simulink model "Leg_4DOF_cT_noise_HGOFeedback"  (R2017a)
settings: Solver=FixedStepAuto  StartTime=0.0  StopTime=4  FixedStep=simulation_step  MaxStep=1e-2  RelTol=1e-3  EnableMultiTasking=on
values from neighbouring files (symbols this model uses):
  Ar = [zeros(4) eye(4); zeros(4) zeros(4)]    [Init_HGO.m]
  beta = 10    [Init_4DOF_cT_noise_HGOFeedback.m]
  BodyContact = [ 4 4 ]    [Init_4DOF_cT_noise_HGOFeedback.m]
  BodyContactPositions = [ contact_point_h, contact_point_t ]    [Init_4DOF_cT_noise_HGOFeedback.m]
  Br = [zeros(4); eye(4)]    [Init_HGO.m]
  Cr = [eye(4) zeros(4)]    [Init_HGO.m]
  dqInit = [ 0 0 0 0 ]'    [Init_4DOF_cT_noise_HGOFeedback.m]
  G = g*ez    [Init_4DOF_cT_noise_HGOFeedback.m]
  G_ctrl = g*ez    [Init_4DOF_cT_noise_HGOFeedback.m]
  h = [ ez -ey -ey -ey ]    [Init_4DOF_cT_noise_HGOFeedback.m]
  h_ctrl = h_ctrl.*param_error    [Init_4DOF_cT_noise_HGOFeedback.m]
  Hmu = [eye(4)/Mu zeros(4); zeros(4) eye(4)/Mu^2]    [Init_HGO.m]
  Inertia = [ I_base I_hip I_thigh I_shin I_foot ]    [Init_4DOF_cT_noise_HGOFeedback.m]
  Inertia_ctrl = Inertia_ctrl.*param_error    [Init_4DOF_cT_noise_HGOFeedback.m]
  joint_type = [ 1 0 0 0 ]    [Init_4DOF_cT_noise_HGOFeedback.m]
  k_b = 5000    [Init_4DOF_cT_noise_HGOFeedback.m]
  Kd = kd*eye(n)    [Init_4DOF_cT_noise_HGOFeedback.m]
  Ki = ki*eye(n)    [Init_4DOF_cT_noise_HGOFeedback.m]
  Kp = kp*eye(n)    [Init_4DOF_cT_noise_HGOFeedback.m]
  L = [ l_base_hip l_hip_thigh l_thigh_shin l_shin_foot ]    [Init_4DOF_cT_noise_HGOFeedback.m]
  L_ctrl = L_ctrl.*param_error    [Init_4DOF_cT_noise_HGOFeedback.m]
  L_hgo = [2*eye(4);6*eye(4)]    [Init_HGO.m]
  Mass = [ mass_base mass_hip mass_thigh mass_shin mass_foot ]    [Init_4DOF_cT_noise_HGOFeedback.m]
  Mass_ctrl = Mass_ctrl.*param_error    [Init_4DOF_cT_noise_HGOFeedback.m]
  qInit = [ 0.0216 0.5675 -0.13 -0.39 ]'    [Init_4DOF_cT_noise_HGOFeedback.m]
  R = [ r_base r_hip r_thigh r_shin r_foot ]    [Init_4DOF_cT_noise_HGOFeedback.m]
  R_ctrl = R_ctrl.*param_error    [Init_4DOF_cT_noise_HGOFeedback.m]
  s_z = 2    [Init_4DOF_cT_noise_HGOFeedback.m]
  simulation_step = 1e-4    (= 0.0001)    [Init_4DOF_cT_noise_HGOFeedback.m]
  step_period = t(end)    [Init_4DOF_cT_noise_HGOFeedback.m]
  tau = 0.001    [Init_4DOF_cT_noise_HGOFeedback.m]
undefined symbols (not defined in the file or in its folder): A, Fstate0, magnitude, offset, w
undefined symbols (not defined in the file): window_size
libraries: simulink x1
settings Model: Creator=Ultron  LastModifiedBy=ignacio
settings DataIOCC: LimitDataPoints=on  SaveFormat=Array
settings OptimizationCC: LifeSpan=inf
settings DebuggingCC: SFUnexpectedBacktrackingDiag=warning  SFNoUnconditionalDefaultTransitionDiag=warning  SFExecutionAtInitializationDiag=none
settings HardwareCC: ProdBitPerPointer=32  ProdBitPerSizeT=32  ProdBitPerPtrDiffT=32  ProdLargestAtomicFloat=None  ProdIntDivRoundTo=Undefined  ProdEndianess=Unspecified  ProdWordSize=32  ProdHWDeviceType=32-bit Generic
settings ModelReferenceCC: PropagateSignalLabelsOutOfModel=off
settings GRTTargetCC: TargetLangStandard=C89/C90 (ANSI)  GeneratePreprocessorConditionals=Disable all
settings ConfigComp: CovMetricSettings=dw  CovHtmlReporting=on  CovSaveCumulativeToWorkspaceVar=on  CovSaveSingleToWorkspaceVar=on  CovExternalEMLEnable=off

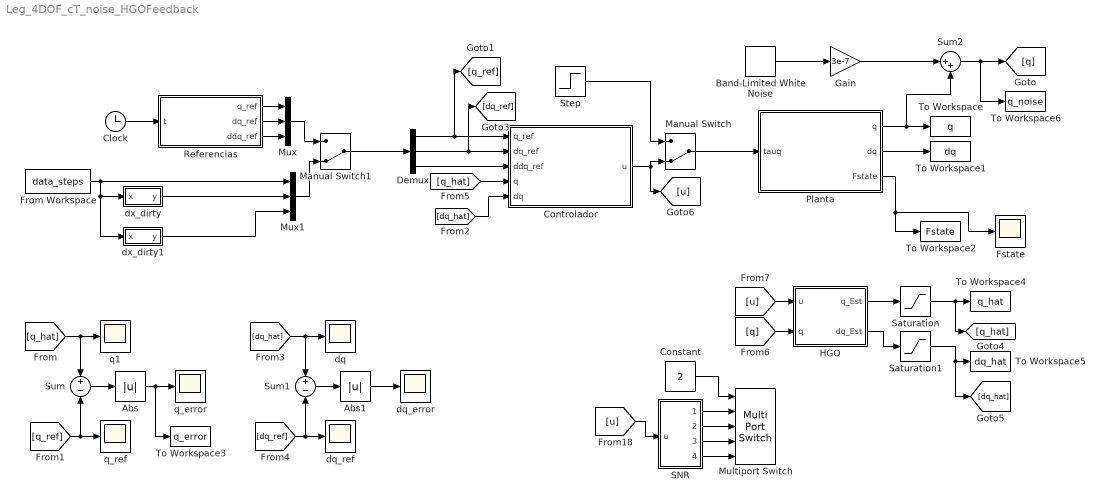
== system Leg_4DOF_cT_noise_HGOFeedback ==
  Abs : Abs
  Abs1 : Abs
  Band-Limited White Noise : simulink/Sources/Band-Limited White Noise  Cov=[0.1]  Ts=simulation_step  seed=[23341]
  Clock : Clock
  Constant : Constant  Value=2
  Controlador : Subsystem
  Demux : Demux  Outputs=3
  From Workspace : FromWorkspace  VariableName=data_steps  SampleTime=0
  Fstate : Scope
  Gain : Gain  Gain=3e-7
  HGO : Subsystem
  Manual Switch : ManualSwitch  CurrentSetting=0
  Manual Switch1 : ManualSwitch  CurrentSetting=0
  Multiport Switch : MultiPortSwitch  Inputs=4
  Mux : Mux  Inputs=3
  Mux1 : Mux  Inputs=3
  Planta : Subsystem
  Referencias : MATLAB Function  TreatAsAtomicUnit=on
  SNR : Subsystem
  Saturation : Saturate  UpperLimit=6*pi  LowerLimit=-6*pi
  Saturation1 : Saturate  UpperLimit=6*pi  LowerLimit=-6*pi
  Step : Step  Before=[0;0;0;0]  After=[0;0;0;0]  SampleTime=0
  Sum : Sum  Inputs=+-
  Sum1 : Sum  Inputs=+-
  Sum2 : Sum  Inputs=|++
  To Workspace : ToWorkspace  VariableName=q  SaveFormat=Timeseries  SampleTime=-1
  To Workspace1 : ToWorkspace  VariableName=dq  SaveFormat=Timeseries  SampleTime=-1
  To Workspace2 : ToWorkspace  VariableName=Fstate  SaveFormat=Timeseries  SampleTime=-1
  To Workspace3 : ToWorkspace  VariableName=q_error  SaveFormat=Timeseries  SampleTime=-1
  To Workspace4 : ToWorkspace  VariableName=q_hat  SaveFormat=Timeseries  SampleTime=-1
  To Workspace5 : ToWorkspace  VariableName=dq_hat  SaveFormat=Timeseries  SampleTime=-1
  To Workspace6 : ToWorkspace  VariableName=q_noise  SaveFormat=Timeseries  SampleTime=-1
  dq : Scope
  dq_error : Scope
  dq_ref : Scope
  dx_dirty : Subsystem
  dx_dirty1 : Subsystem
  q1 : Scope
  q_error : Scope
  q_ref : Scope
  wires:
  Planta/2(dq) -> To Workspace1/1
  Manual Switch/1 -> Planta/1(tauq)
  Step/1 -> Manual Switch/1
  Clock/1 -> Referencias/1(t)
  Planta/1(q) -> Sum2/2, To Workspace/1
  Planta/3(Fstate) -> To Workspace2/1, Fstate/1
  Referencias/1(q_ref) -> Mux/1
  Referencias/2(dq_ref) -> Mux/2
  Referencias/3(ddq_ref) -> Mux/3
  From Workspace/1 -> dx_dirty1/1(x), dx_dirty/1(x), Mux1/1
  dx_dirty/1(y) -> Mux1/2
  dx_dirty1/1(y) -> Mux1/3
  Mux/1 -> Manual Switch1/1
  Mux1/1 -> Manual Switch1/2
  Manual Switch1/1 -> Demux/1
  Demux/1 -> [q_ref], Controlador/1(q_ref)
  Demux/2 -> [dq_ref], Controlador/2(dq_ref)
  Demux/3 -> Controlador/3(ddq_ref)
  [q_hat] -> q1/1, Sum/1
  [q_ref] -> q_ref/1, Sum/2
  Sum/1 -> Abs/1
  Abs/1 -> To Workspace3/1, q_error/1
  [q_hat] -> Controlador/4(q)
  [dq_ref] -> dq_ref/1, Sum1/2
  Sum1/1 -> Abs1/1
  Abs1/1 -> dq_error/1
  [dq_hat] -> dq/1, Sum1/1
  [dq_hat] -> Controlador/5(dq)
  Controlador/1(u) -> [u], Manual Switch/2
  Saturation/1 -> [q_hat], To Workspace4/1
  HGO/1(q_Est) -> Saturation/1
  [q] -> HGO/2(q)
  HGO/2(dq_Est) -> Saturation1/1
  Saturation1/1 -> [dq_hat], To Workspace5/1
  [u] -> HGO/1(u)
  Sum2/1 -> To Workspace6/1, [q]
  Band-Limited White Noise/1 -> Gain/1
  Gain/1 -> Sum2/1
  [u] -> SNR/1(u)
  SNR/1(Out1) -> Multiport Switch/2
  SNR/2(Out2) -> Multiport Switch/3
  SNR/3(Out5) -> Multiport Switch/4
  SNR/4(Out3) -> Multiport Switch/5
  Constant/1 -> Multiport Switch/1

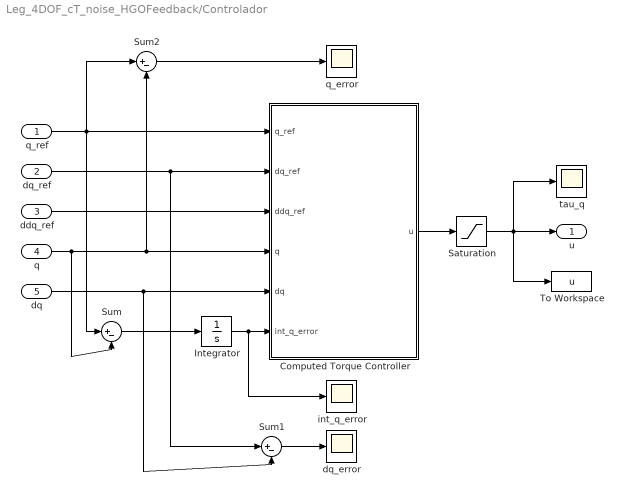
== system Leg_4DOF_cT_noise_HGOFeedback/Controlador ==
  q_ref : Inport
  dq_ref : Inport  Port=2
  ddq_ref : Inport  Port=3
  q : Inport  Port=4
  dq : Inport  Port=5
  Computed Torque Controller : MATLAB Function  TreatAsAtomicUnit=on
  Integrator : Integrator  InitialCondition=zeros(4,1)
  Saturation : Saturate  UpperLimit=800  LowerLimit=-800
  Sum : Sum  Inputs=|+-
  Sum1 : Sum  Inputs=|+-
  Sum2 : Sum  Inputs=|+-
  To Workspace : ToWorkspace  VariableName=u  SaveFormat=Timeseries  SampleTime=-1
  dq_error : Scope
  int_q_error : Scope
  q_error : Scope
  tau_q : Scope
  u : Outport
  wires:
  Computed Torque Controller/1(u) -> Saturation/1
  q_ref/1 -> Sum2/1, Sum/1, Computed Torque Controller/1(q_ref)
  dq_ref/1 -> Sum1/1, Computed Torque Controller/2(dq_ref)
  q/1 -> Sum/2, Computed Torque Controller/4(q), Sum2/2
  Sum1/1 -> dq_error/1
  ddq_ref/1 -> Computed Torque Controller/3(ddq_ref)
  dq/1 -> Sum1/2, Computed Torque Controller/5(dq)
  Sum/1 -> Integrator/1
  Integrator/1 -> int_q_error/1, Computed Torque Controller/6(int_q_error)
  Sum2/1 -> q_error/1
  Saturation/1 -> To Workspace/1, tau_q/1, u/1

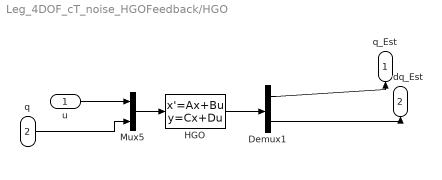
== system Leg_4DOF_cT_noise_HGOFeedback/HGO ==
  u : Inport
  q : Inport  Port=2
  Demux1 : Demux  Outputs=2
  HGO : StateSpace  A=Ar-Hmu*L_hgo*Cr  B=[Br Hmu*L_hgo]  C=eye(8)  D=zeros(8)  X0=[qInit; dqInit]
  Mux5 : Mux  Inputs=2
  q_Est : Outport  PortDimensions=4
  dq_Est : Outport  Port=2  PortDimensions=4
  wires:
  Mux5/1 -> HGO/1
  Demux1/1 -> q_Est/1
  Demux1/2 -> dq_Est/1
  u/1 -> Mux5/1
  q/1 -> Mux5/2
  HGO/1 -> Demux1/1

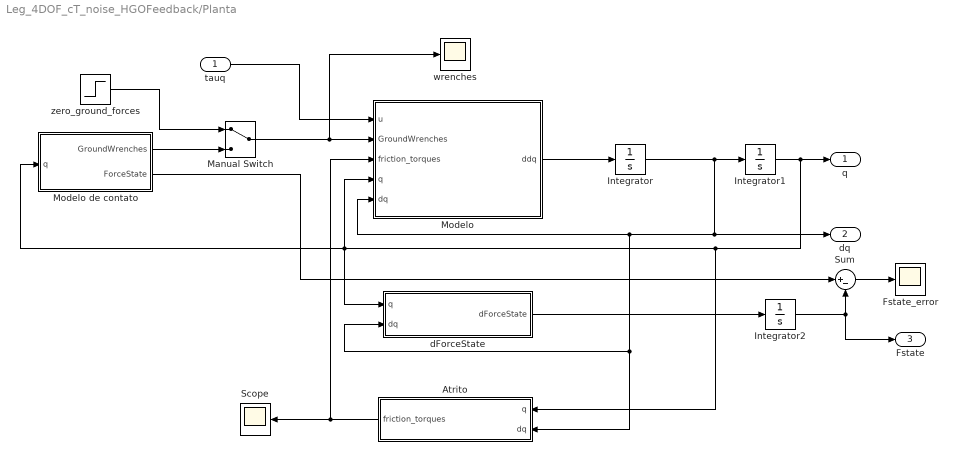
== system Leg_4DOF_cT_noise_HGOFeedback/Planta ==
  tauq : Inport
  Atrito : MATLAB Function  TreatAsAtomicUnit=on
  Fstate_error : Scope
  Integrator : Integrator  InitialCondition=dqInit
  Integrator1 : Integrator  InitialCondition=qInit
  Integrator2 : Integrator  InitialCondition=Fstate0
  Manual Switch : ManualSwitch
  Modelo : MATLAB Function  TreatAsAtomicUnit=on
  Modelo de contato : MATLAB Function  TreatAsAtomicUnit=on
  Scope : Scope
  Sum : Sum  Inputs=|+-
  dForceState : MATLAB Function  TreatAsAtomicUnit=on
  wrenches : Scope
  zero_ground_forces : Step  Before=zeros(6,2)  After=zeros(6,2)  SampleTime=0
  q : Outport
  dq : Outport  Port=2
  Fstate : Outport  Port=3
  wires:
  Integrator1/1 -> dForceState/1(q), Modelo de contato/1(q), Modelo/4(q), Atrito/1(q), q/1
  Integrator/1 -> Integrator1/1, Modelo/5(dq), dForceState/2(dq), Atrito/2(dq), dq/1
  Atrito/1(friction_torques) -> Modelo/3(friction_torques), Scope/1
  tauq/1 -> Modelo/1(u)
  Integrator2/1 -> Sum/2, Fstate/1
  dForceState/1(dForceState) -> Integrator2/1
  Modelo de contato/2(ForceState) -> Sum/1
  Sum/1 -> Fstate_error/1
  Manual Switch/1 -> wrenches/1, Modelo/2(GroundWrenches)
  Modelo de contato/1(GroundWrenches) -> Manual Switch/2
  zero_ground_forces/1 -> Manual Switch/1
  Modelo/1(ddq) -> Integrator/1

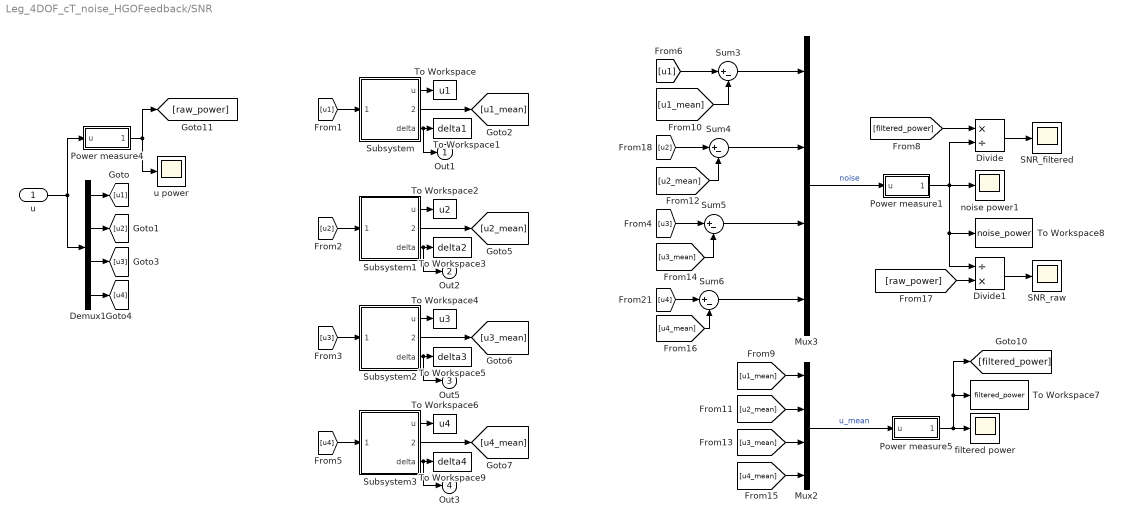
== system Leg_4DOF_cT_noise_HGOFeedback/SNR ==
  u : Inport
  Demux1 : Demux
  Divide : Product  Inputs=*/
  Divide1 : Product  Inputs=/*
  Mux2 : Mux
  Mux3 : Mux
  Power measure1 : Subsystem  mask(Measure power){window=0.001, sampling=1e-3}
      mask prompts: window "Window Length"
      mask help: Foo bar
      mask init:
      | global step_period;
      | 
      | N = step_period / window;
  Power measure4 : Subsystem  mask(Measure power){window=0.001, sampling=1e-3}
      mask prompts: window "Window Length"
      mask help: Foo bar
      mask init:
      | global step_period;
      | 
      | N = step_period / window;
  Power measure5 : Subsystem  mask(Measure power){window=0.001, sampling=1e-3}
      mask prompts: window "Window Length"
      mask help: Foo bar
      mask init:
      | global step_period;
      | 
      | N = step_period / window;
  SNR_filtered : Scope
  SNR_raw : Scope
  Subsystem : Subsystem  mask{N=window_size(1)}
      mask prompts: N "Window size"
  Subsystem1 : Subsystem  mask{N=window_size(2)}
      mask prompts: N "Window size"
  Subsystem2 : Subsystem  mask{N=window_size(3)}
      mask prompts: N "Window size"
  Subsystem3 : Subsystem  mask{N=window_size(4)}
      mask prompts: N "Window size"
  Sum{3..6} (4 alike) : Sum  Inputs=|+-
  To Workspace : ToWorkspace  VariableName=u1  SaveFormat=Timeseries  SampleTime=-1
  To Workspace1 : ToWorkspace  VariableName=delta1  SaveFormat=Timeseries  SampleTime=-1
  To Workspace2 : ToWorkspace  VariableName=u2  SaveFormat=Timeseries  SampleTime=-1
  To Workspace3 : ToWorkspace  VariableName=delta2  SaveFormat=Timeseries  SampleTime=-1
  To Workspace4 : ToWorkspace  VariableName=u3  SaveFormat=Timeseries  SampleTime=-1
  To Workspace5 : ToWorkspace  VariableName=delta3  SaveFormat=Timeseries  SampleTime=-1
  To Workspace6 : ToWorkspace  VariableName=u4  SaveFormat=Timeseries  SampleTime=-1
  To Workspace7 : ToWorkspace  VariableName=filtered_power  SaveFormat=Timeseries  SampleTime=-1
  To Workspace8 : ToWorkspace  VariableName=noise_power  SaveFormat=Timeseries  SampleTime=-1
  To Workspace9 : ToWorkspace  VariableName=delta4  SaveFormat=Timeseries  SampleTime=-1
  filtered power : Scope
  noise power1 : Scope
  u power : Scope
  Out1 : Outport
  Out2 : Outport  Port=2
  Out5 : Outport  Port=3
  Out3 : Outport  Port=4
  wires:
  Sum6/1 -> Mux3/4
  Power measure5/1(Power) -> [filtered_power], To Workspace7/1, filtered power/1
  [u1_mean] -> Sum3/2
  Subsystem/2(mean) -> [u1_mean]
  [u4_mean] -> Sum6/2
  u/1 -> Power measure4/1(u), Demux1/1
  Divide1/1 -> SNR_raw/1
  [u1_mean] -> Mux2/1
  Subsystem/1(u) -> To Workspace/1
  Divide/1 -> SNR_filtered/1
  [u3_mean] -> Mux2/3
  Mux3/1 -> Power measure1/1(u)  "noise"
  [u4_mean] -> Mux2/4
  Sum5/1 -> Mux3/3
  [filtered_power] -> Divide/1
  Power measure1/1(Power) -> To Workspace8/1, Divide1/1, Divide/2, noise power1/1
  Mux2/1 -> Power measure5/1(u)  "u_mean"
  Power measure4/1(Power) -> [raw_power], u power/1
  Sum3/1 -> Mux3/1
  [u2_mean] -> Sum4/2
  [u3_mean] -> Sum5/2
  [raw_power] -> Divide1/2
  Sum4/1 -> Mux3/2
  [u2_mean] -> Mux2/2
  Subsystem/3(delta) -> Out1/1, To Workspace1/1
  Demux1/1 -> [u1]
  [u1] -> Subsystem/1(signal)
  [u1] -> Sum3/1
  Demux1/2 -> [u2]
  [u2] -> Sum4/1
  Demux1/3 -> [u3]
  [u3] -> Sum5/1
  Demux1/4 -> [u4]
  [u4] -> Sum6/1
  [u2] -> Subsystem1/1(signal)
  Subsystem1/2(mean) -> [u2_mean]
  Subsystem1/1(u) -> To Workspace2/1
  Subsystem1/3(delta) -> Out2/1, To Workspace3/1
  [u3] -> Subsystem2/1(signal)
  Subsystem2/2(mean) -> [u3_mean]
  Subsystem2/1(u) -> To Workspace4/1
  Subsystem2/3(delta) -> Out5/1, To Workspace5/1
  [u4] -> Subsystem3/1(signal)
  Subsystem3/2(mean) -> [u4_mean]
  Subsystem3/1(u) -> To Workspace6/1
  Subsystem3/3(delta) -> Out3/1, To Workspace9/1

== system Leg_4DOF_cT_noise_HGOFeedback/dx_dirty ==
  x : Inport
  Gain : Gain  Gain=1/tau
  Gain1 : Gain  Gain=1/tau
  Integrator : Integrator  InitialCondition=dqInit
  Sum : Sum  Inputs=|--
  Sum1 : Sum  Inputs=++|
  y : Outport
  wires:
  Gain1/1 -> Sum1/1, Sum/1
  x/1 -> Gain1/1
  Gain/1 -> Integrator/1
  Integrator/1 -> Sum/2, Sum1/2
  Sum/1 -> Gain/1
  Sum1/1 -> y/1

== system Leg_4DOF_cT_noise_HGOFeedback/dx_dirty1 ==
  x : Inport
  Gain : Gain  Gain=1/tau
  Gain1 : Gain  Gain=1/tau
  Integrator : Integrator  InitialCondition=zeros(4,1)
  Sum : Sum  Inputs=|--
  Sum1 : Sum  Inputs=++|
  y : Outport
  wires:
  Sum1/1 -> y/1
  Sum/1 -> Gain/1
  Integrator/1 -> Sum1/2, Sum/2
  Gain/1 -> Integrator/1
  x/1 -> Gain1/1
  Gain1/1 -> Sum/1, Sum1/1

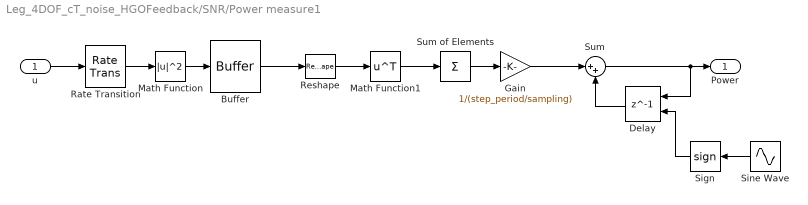
== system Leg_4DOF_cT_noise_HGOFeedback/SNR/Power measure1 ==
  u : Inport
  Buffer : Buffer  N=4* window/sampling  OutputFrames=off
  Delay : Delay  DelayLength=1  ExternalReset=Either
      settings: InputPortMap=u0,r5
  Gain : Gain  Gain=1/(step_period/sampling)
  Math Function : Math  Operator=magnitude^2  SaturateOnIntegerOverflow=on
  Math Function1 : Math  Operator=transpose  SaturateOnIntegerOverflow=on
  Rate Transition : RateTransition  OutPortSampleTime=sampling
  Reshape : Reshape  OutputDimensionality=Customize  OutputDimensions=[4,window/sampling]
  Sign : Signum
  Sine Wave : Sin  Frequency=2*pi / (2 * step_period)  SampleTime=window
  Sum : Sum  Inputs=|++
  Sum of Elements : Sum  Inputs=+  CollapseMode=Specified dimension
  Power : Outport
  wires:
  u/1 -> Rate Transition/1
  Sign/1 -> Delay/2
  Sine Wave/1 -> Sign/1
  Delay/1 -> Sum/2
  Sum/1 -> Power/1, Delay/1
  Math Function1/1 -> Sum of Elements/1
  Buffer/1 -> Reshape/1
  Sum of Elements/1 -> Gain/1
  Reshape/1 -> Math Function1/1
  Gain/1 -> Sum/1
  Rate Transition/1 -> Math Function/1
  Math Function/1 -> Buffer/1

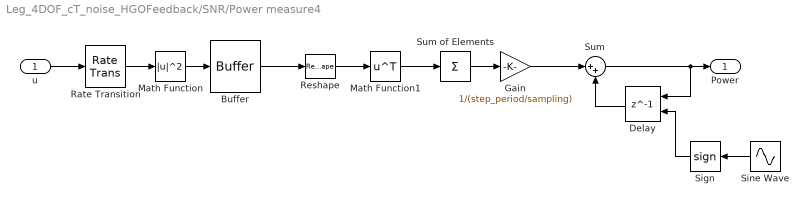
== system Leg_4DOF_cT_noise_HGOFeedback/SNR/Power measure4 ==
  u : Inport
  Buffer : Buffer  N=4* window/sampling  OutputFrames=off
  Delay : Delay  DelayLength=1  ExternalReset=Either
      settings: InputPortMap=u0,r5
  Gain : Gain  Gain=1/(step_period/sampling)
  Math Function : Math  Operator=magnitude^2  SaturateOnIntegerOverflow=on
  Math Function1 : Math  Operator=transpose  SaturateOnIntegerOverflow=on
  Rate Transition : RateTransition  OutPortSampleTime=sampling
  Reshape : Reshape  OutputDimensionality=Customize  OutputDimensions=[4,window/sampling]
  Sign : Signum
  Sine Wave : Sin  Frequency=2*pi / (2 * step_period)  SampleTime=window
  Sum : Sum  Inputs=|++
  Sum of Elements : Sum  Inputs=+  CollapseMode=Specified dimension
  Power : Outport
  wires:
  u/1 -> Rate Transition/1
  Sign/1 -> Delay/2
  Sine Wave/1 -> Sign/1
  Delay/1 -> Sum/2
  Sum/1 -> Power/1, Delay/1
  Math Function1/1 -> Sum of Elements/1
  Buffer/1 -> Reshape/1
  Sum of Elements/1 -> Gain/1
  Reshape/1 -> Math Function1/1
  Gain/1 -> Sum/1
  Rate Transition/1 -> Math Function/1
  Math Function/1 -> Buffer/1

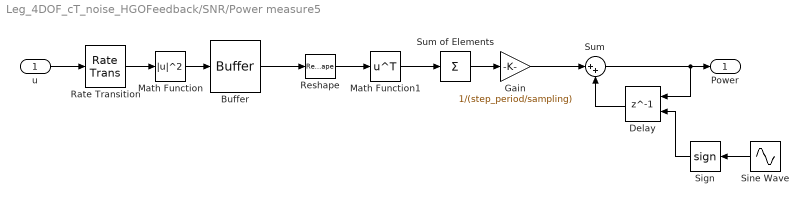
== system Leg_4DOF_cT_noise_HGOFeedback/SNR/Power measure5 ==
  u : Inport
  Buffer : Buffer  N=4* window/sampling  OutputFrames=off
  Delay : Delay  DelayLength=1  ExternalReset=Either
      settings: InputPortMap=u0,r5
  Gain : Gain  Gain=1/(step_period/sampling)
  Math Function : Math  Operator=magnitude^2  SaturateOnIntegerOverflow=on
  Math Function1 : Math  Operator=transpose  SaturateOnIntegerOverflow=on
  Rate Transition : RateTransition  OutPortSampleTime=sampling
  Reshape : Reshape  OutputDimensionality=Customize  OutputDimensions=[4,window/sampling]
  Sign : Signum
  Sine Wave : Sin  Frequency=2*pi / (2 * step_period)  SampleTime=window
  Sum : Sum  Inputs=|++
  Sum of Elements : Sum  Inputs=+  CollapseMode=Specified dimension
  Power : Outport
  wires:
  Math Function/1 -> Buffer/1
  Rate Transition/1 -> Math Function/1
  Gain/1 -> Sum/1
  Reshape/1 -> Math Function1/1
  Sum of Elements/1 -> Gain/1
  Buffer/1 -> Reshape/1
  Math Function1/1 -> Sum of Elements/1
  Sum/1 -> Delay/1, Power/1
  Delay/1 -> Sum/2
  Sine Wave/1 -> Sign/1
  Sign/1 -> Delay/2
  u/1 -> Rate Transition/1

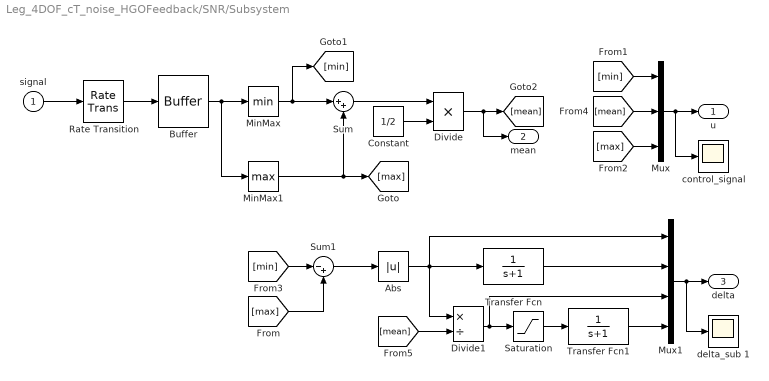
== system Leg_4DOF_cT_noise_HGOFeedback/SNR/Subsystem ==
  signal : Inport
  Abs : Abs
  Buffer : Buffer  N=N  V=N - 1  OutputFrames=off
  Constant : Constant  Value=1/2
  Divide : Product  SaturateOnIntegerOverflow=on  RndMeth=Zero
  Divide1 : Product  Inputs=*/  SaturateOnIntegerOverflow=on  RndMeth=Zero
  MinMax : MinMax
  MinMax1 : MinMax  Function=max
  Mux : Mux  Inputs=3
  Mux1 : Mux
  Rate Transition : RateTransition  OutPortSampleTime=simulation_step
  Saturation : Saturate  UpperLimit=800  LowerLimit=-800
  Sum : Sum  Inputs=|++
  Sum1 : Sum  Inputs=|-+
  Transfer Fcn : TransferFcn  Denominator=[1 1]
  Transfer Fcn1 : TransferFcn  Denominator=[1 1]
  control_signal : Scope
  delta_sub 1 : Scope
  u : Outport
  mean : Outport  Port=2
  delta : Outport  Port=3
  wires:
  MinMax1/1 -> Sum/2, [max]
  signal/1 -> Rate Transition/1
  MinMax/1 -> [min], Sum/1
  Sum/1 -> Divide/1
  Rate Transition/1 -> Buffer/1
  Constant/1 -> Divide/2
  Buffer/1 -> MinMax1/1, MinMax/1
  Sum1/1 -> Abs/1
  Abs/1 -> Mux1/1, Divide1/1, Transfer Fcn/1
  Divide1/1 -> Saturation/1, Mux1/3
  [min] -> Mux/1
  [max] -> Mux/3
  [max] -> Sum1/2
  [min] -> Sum1/1
  Divide/1 -> mean/1, [mean]
  [mean] -> Mux/2
  Mux/1 -> control_signal/1, u/1
  [mean] -> Divide1/2
  Transfer Fcn/1 -> Mux1/2
  Transfer Fcn1/1 -> Mux1/4
  Mux1/1 -> delta_sub 1/1, delta/1
  Saturation/1 -> Transfer Fcn1/1

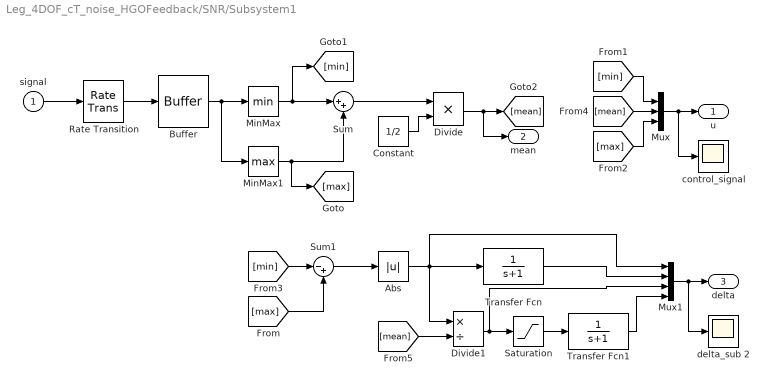
== system Leg_4DOF_cT_noise_HGOFeedback/SNR/Subsystem1 ==
  signal : Inport
  Abs : Abs
  Buffer : Buffer  N=N  V=N - 1  OutputFrames=off
  Constant : Constant  Value=1/2
  Divide : Product  SaturateOnIntegerOverflow=on  RndMeth=Zero
  Divide1 : Product  Inputs=*/  SaturateOnIntegerOverflow=on  RndMeth=Zero
  MinMax : MinMax
  MinMax1 : MinMax  Function=max
  Mux : Mux  Inputs=3
  Mux1 : Mux
  Rate Transition : RateTransition  OutPortSampleTime=simulation_step
  Saturation : Saturate  UpperLimit=800  LowerLimit=-800
  Sum : Sum  Inputs=|++
  Sum1 : Sum  Inputs=|-+
  Transfer Fcn : TransferFcn  Denominator=[1 1]
  Transfer Fcn1 : TransferFcn  Denominator=[1 1]
  control_signal : Scope
  delta_sub 2 : Scope
  u : Outport
  mean : Outport  Port=2
  delta : Outport  Port=3
  wires:
  MinMax1/1 -> Sum/2, [max]
  signal/1 -> Rate Transition/1
  MinMax/1 -> [min], Sum/1
  Sum/1 -> Divide/1
  Rate Transition/1 -> Buffer/1
  Constant/1 -> Divide/2
  Buffer/1 -> MinMax1/1, MinMax/1
  Sum1/1 -> Abs/1
  Abs/1 -> Mux1/1, Divide1/1, Transfer Fcn/1
  Divide1/1 -> Saturation/1, Mux1/3
  [min] -> Mux/1
  [max] -> Mux/3
  [max] -> Sum1/2
  [min] -> Sum1/1
  Divide/1 -> mean/1, [mean]
  [mean] -> Mux/2
  Mux/1 -> control_signal/1, u/1
  [mean] -> Divide1/2
  Transfer Fcn/1 -> Mux1/2
  Transfer Fcn1/1 -> Mux1/4
  Mux1/1 -> delta_sub 2/1, delta/1
  Saturation/1 -> Transfer Fcn1/1

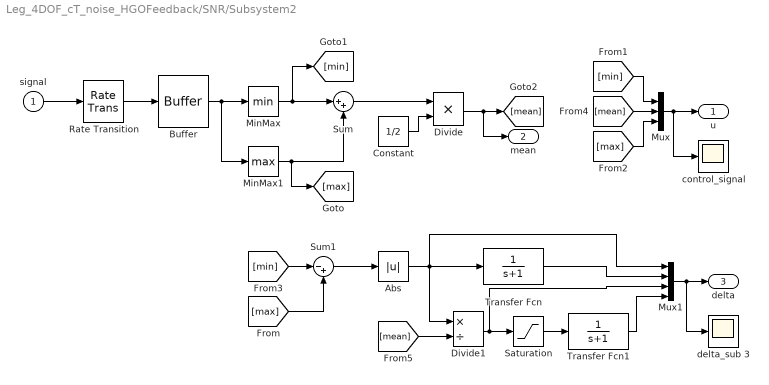
== system Leg_4DOF_cT_noise_HGOFeedback/SNR/Subsystem2 ==
  signal : Inport
  Abs : Abs
  Buffer : Buffer  N=N  V=N - 1  OutputFrames=off
  Constant : Constant  Value=1/2
  Divide : Product  SaturateOnIntegerOverflow=on  RndMeth=Zero
  Divide1 : Product  Inputs=*/  SaturateOnIntegerOverflow=on  RndMeth=Zero
  MinMax : MinMax
  MinMax1 : MinMax  Function=max
  Mux : Mux  Inputs=3
  Mux1 : Mux
  Rate Transition : RateTransition  OutPortSampleTime=simulation_step
  Saturation : Saturate  UpperLimit=800  LowerLimit=-800
  Sum : Sum  Inputs=|++
  Sum1 : Sum  Inputs=|-+
  Transfer Fcn : TransferFcn  Denominator=[1 1]
  Transfer Fcn1 : TransferFcn  Denominator=[1 1]
  control_signal : Scope
  delta_sub 3 : Scope
  u : Outport
  mean : Outport  Port=2
  delta : Outport  Port=3
  wires:
  MinMax1/1 -> Sum/2, [max]
  signal/1 -> Rate Transition/1
  MinMax/1 -> [min], Sum/1
  Sum/1 -> Divide/1
  Rate Transition/1 -> Buffer/1
  Constant/1 -> Divide/2
  Buffer/1 -> MinMax1/1, MinMax/1
  Sum1/1 -> Abs/1
  Abs/1 -> Mux1/1, Divide1/1, Transfer Fcn/1
  Divide1/1 -> Saturation/1, Mux1/3
  [min] -> Mux/1
  [max] -> Mux/3
  [max] -> Sum1/2
  [min] -> Sum1/1
  Divide/1 -> mean/1, [mean]
  [mean] -> Mux/2
  Mux/1 -> control_signal/1, u/1
  [mean] -> Divide1/2
  Transfer Fcn/1 -> Mux1/2
  Transfer Fcn1/1 -> Mux1/4
  Mux1/1 -> delta_sub 3/1, delta/1
  Saturation/1 -> Transfer Fcn1/1

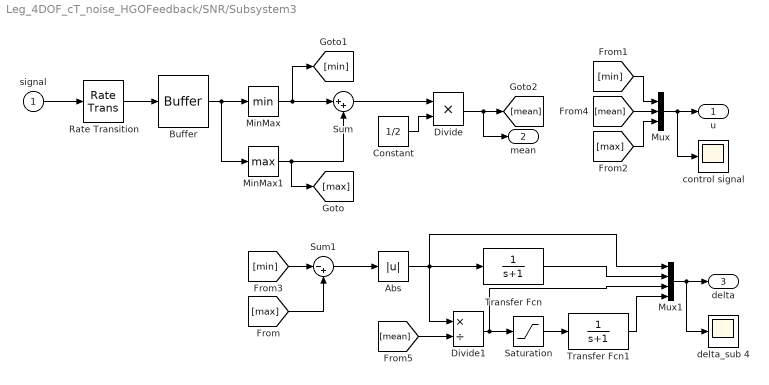
== system Leg_4DOF_cT_noise_HGOFeedback/SNR/Subsystem3 ==
  signal : Inport
  Abs : Abs
  Buffer : Buffer  N=N  V=N - 1  OutputFrames=off
  Constant : Constant  Value=1/2
  Divide : Product  SaturateOnIntegerOverflow=on  RndMeth=Zero
  Divide1 : Product  Inputs=*/  SaturateOnIntegerOverflow=on  RndMeth=Zero
  MinMax : MinMax
  MinMax1 : MinMax  Function=max
  Mux : Mux  Inputs=3
  Mux1 : Mux
  Rate Transition : RateTransition  OutPortSampleTime=simulation_step
  Saturation : Saturate  UpperLimit=800  LowerLimit=-800
  Sum : Sum  Inputs=|++
  Sum1 : Sum  Inputs=|-+
  Transfer Fcn : TransferFcn  Denominator=[1 1]
  Transfer Fcn1 : TransferFcn  Denominator=[1 1]
  control signal : Scope
  delta_sub 4 : Scope
  u : Outport
  mean : Outport  Port=2
  delta : Outport  Port=3
  wires:
  MinMax1/1 -> Sum/2, [max]
  signal/1 -> Rate Transition/1
  MinMax/1 -> [min], Sum/1
  Sum/1 -> Divide/1
  Rate Transition/1 -> Buffer/1
  Constant/1 -> Divide/2
  Buffer/1 -> MinMax1/1, MinMax/1
  Sum1/1 -> Abs/1
  Abs/1 -> Mux1/1, Divide1/1, Transfer Fcn/1
  Divide1/1 -> Saturation/1, Mux1/3
  [min] -> Mux/1
  [max] -> Mux/3
  [max] -> Sum1/2
  [min] -> Sum1/1
  Divide/1 -> mean/1, [mean]
  [mean] -> Mux/2
  Mux/1 -> control signal/1, u/1
  [mean] -> Divide1/2
  Transfer Fcn/1 -> Mux1/2
  Transfer Fcn1/1 -> Mux1/4
  Mux1/1 -> delta_sub 4/1, delta/1
  Saturation/1 -> Transfer Fcn1/1

== matlab function Leg_4DOF_cT_noise_HGOFeedback/Controlador/Computed Torque Controller ==
  data: q_ref input; dq_ref input; ddq_ref input; u output; q input; dq input; int_q_error input; joint_type parameter; Mass_ctrl parameter; Inertia_ctrl parameter; R_ctrl parameter; L_ctrl parameter; h_ctrl parameter; G_ctrl parameter; Kp parameter; Kd parameter; Ki parameter
function u = fcn(q_ref, dq_ref, ddq_ref, q, dq, int_q_error, joint_type, Mass_ctrl, Inertia_ctrl, R_ctrl, L_ctrl, h_ctrl, G_ctrl, Kp, Kd, Ki )
%% Prostectics control

v = ddq_ref + Kd*(dq_ref - dq) + Kp*(q_ref - q) + Ki*int_q_error;
u = prosthetics_inverse_dynamics( q, dq, v, joint_type, Mass_ctrl, Inertia_ctrl, R_ctrl, L_ctrl, h_ctrl, G_ctrl );

== matlab function Leg_4DOF_cT_noise_HGOFeedback/Planta/Modelo ==
  data: u input; GroundWrenches input; friction_torques input; q input; dq input; joint_type parameter; Mass parameter; Inertia parameter; R parameter; L parameter; h parameter; G parameter; ddq output; BodyContactPositions parameter; BodyContact parameter
function ddq = fcn( u, GroundWrenches, friction_torques, q, dq, joint_type, Mass, Inertia, R, L, h, G, BodyContactPositions,  BodyContact )
% direct dynamics

% n = length(q);

% coder.extrinsic('model_prosthetics_mex');
% ddq = coder.nullcopy(zeros(n,1));
% Friction_torques = coder.nullcopy(zeros(n,1));

ddq = model_prosthetics( u, q, dq, joint_type, Mass, Inertia, R, L, h, G, friction_torques, BodyContact, GroundWrenches, BodyContactPositions );
% ddq = model_prosthetics_mex( u, q, dq, joint_type, Mass, Inertia, R, L, h, G, friction_coefs, BodyContact, BodyContactWrenches, BodyContactPositions );

== matlab function Leg_4DOF_cT_noise_HGOFeedback/Referencias ==
  data: t input; q_ref output; dq_ref output; ddq_ref output; A parameter; offset parameter; w parameter
function [ q_ref, dq_ref, ddq_ref ] = fcn( t, A, offset, w)
% generate reference

% q_ref = A*sin(w*t + offset);
% dq_ref = A*w*cos(w*t + offset);
% ddq_ref = -A*(w^2)*sin(w*t + offset);

q_ref = zeros(4,1);
dq_ref = zeros(4,1);
ddq_ref = zeros(4,1);

for i = 1:4
    q_ref(i) = A(i)*sin(w(i)*t + offset(i));
    dq_ref(i) = A(i)*w(i)*cos(w(i)*t + offset(i));
    ddq_ref(i) = -A(i)*(w(i)^2)*sin(w(i)*t + offset(i));
end

== matlab function Leg_4DOF_cT_noise_HGOFeedback/Planta/Atrito ==
  data: friction_torques output; q input; dq input
function friction_torques = fcn( q, dq )
%% Joint friction model
n = length(q);
friction_torques = zeros(n,1);

== matlab function Leg_4DOF_cT_noise_HGOFeedback/Planta/Modelo de contato ==
  data: GroundWrenches output; q input; BodyContactPositions parameter; s_z parameter; L parameter; h parameter; beta parameter; k_b parameter; joint_type parameter; ForceState output
function [ GroundWrenches, ForceState ] = fcn( q, BodyContactPositions, s_z, L, h, beta,  k_b, joint_type )
% function BodyContactWrenches = fcn( t, q, L, h, BodyContactPositions, joint_type, sz, beta, kb)
% Esta função calcula as forças de contato com o chão

[ GroundWrenches, ForceState ] = ground_model( q, BodyContactPositions, s_z, L, h, beta,  k_b, joint_type );

== matlab function Leg_4DOF_cT_noise_HGOFeedback/Planta/dForceState ==
  data: q input; dq input; dForceState output; L parameter; h parameter; joint_type parameter; BodyContactPositions parameter; s_z parameter; beta parameter; k_b parameter
function dForceState = fcn( q, dq, L, h, joint_type,  BodyContactPositions, s_z, beta, k_b)
%% Dinâmica do modelo de contato (em coordenadas inerciais)

%% Computes the velocity body twist of the given point.
body = 4;
contact_point_h = BodyContactPositions(:,1);
contact_point_t = BodyContactPositions(:,2);
V_h = prosthetics_diff_kinematics( q, dq, L, h, body, contact_point_h, joint_type );
V_t = prosthetics_diff_kinematics( q, dq, L, h, body, contact_point_t, joint_type );

%% Computes 
[ P_h, R_h ] = prosthetics_forward_kinematics( q, L, h, body, contact_point_h, joint_type );
[ P_t, R_t ] = prosthetics_forward_kinematics( q, L, h, body, contact_point_h, joint_type );
z_h = P_h(3);
z_t = P_t(3);

%% Converts body linear velocity into inertial velocty
v_h = R_h*V_h(1:3);
v_t = R_t*V_t(1:3);

dz_h = v_h(3);
dz_t = v_t(3);

dF_zh = -(k_b/2)*dz_h*(1+sign(z_h - s_z));
dF_zt = -(k_b/2)*dz_t*(1+sign(z_t - s_z));

dF_xh = beta*dF_zh;
dF_xt = beta*dF_zt;

dForceState = [ dF_zh dF_zt dF_xh dF_xt ]';
